simulink model "EPT"  (R2019b)
settings: Solver=FixedStepDiscrete  StartTime=0.0  StopTime=5  FixedStep=0.005  RelTol=1e-3  EnableMultiTasking=on
PreLoadFcn:
  | try, model_open; catch, disp('Error occurred while executing model pre-load callback: model_open.m'); disp('Please assure that the MATLAB working directory is set to the model directory before opening.'); end
InitFcn:
  | try, model_open; catch, end
undefined symbols (not defined in the file or in its folder): Bridge, GCM, H, ln, raptor_get_param_eval, raptor_get_safe_string, raptor_xcp_function
libraries: Raptor_lib x2810, simulink x374, hdlsllib x19
(part 3 of 45)

== system EPT/Foreground_TimeBase_5ms/CHG//DCHG_PW_Control/Batt_Temperature Coefficient ==
  Compare To Constant : simulink/Logic and Bit Operations/Compare To Constant  relop=<  const=20  OutDataTypeStr=boolean
  Compare To Constant1 : simulink/Logic and Bit Operations/Compare To Constant  relop=<  const=35  OutDataTypeStr=boolean
  Constant4 : Constant
  Constant5 : Constant
  Demux1 : Demux  Outputs=2
  Max : MinMax  Function=max  Inputs=2
  MinMax : MinMax  Inputs=2
  Mux1 : Mux  Inputs=2
  Product1 : Product
  Saturation : Saturate  UpperLimit=60  LowerLimit=-10
  Saturation1 : Saturate  UpperLimit=60  LowerLimit=-10
  Switch : Switch  Criteria=u2 > Threshold
  Switch1 : Switch  Criteria=u2 > Threshold
  raptor_data_def1 : Raptor_lib/Data Storage/raptor_data_def  dataName='Max_CellT'  initValue=0  dataType=double  storage=Volatile (RAM)  calVisible=on  calType=Measurement  calDispType=Number  calEnum={'False', 'True'}  calGain=1.0  calOffset=0  calMin=-inf  calMax=inf  calFormat='-1'  calUnit=''  calHelp=''  calAccess=1  calFunction=raptor_xcp_function(gcb)  calDispHeaders=off  calColHeaders={'Col1' 'Col2' 'Col3'}  calRowHeaders={'Row1' 'Row2' 'Row3'}
      settings: SourceProductName=Raptor
  raptor_data_def2 : Raptor_lib/Data Storage/raptor_data_def  dataName='Min_CellT'  initValue=0  dataType=double  storage=Volatile (RAM)  calVisible=on  calType=Measurement  calDispType=Number  calEnum={'False', 'True'}  calGain=1.0  calOffset=0  calMin=-inf  calMax=inf  calFormat='-1'  calUnit=''  calHelp=''  calAccess=1  calFunction=raptor_xcp_function(gcb)  calDispHeaders=off  calColHeaders={'Col1' 'Col2' 'Col3'}  calRowHeaders={'Row1' 'Row2' 'Row3'}
      settings: SourceProductName=Raptor
  raptor_data_read1 : Raptor_lib/Data Storage/raptor_data_read  dataName='CMU1_CELL_TEMP_MIN'  dataShape=Scalar  idxSource=Input  idxRow=1  idxCol=1
      settings: SourceProductName=Raptor
  raptor_data_read2 : Raptor_lib/Data Storage/raptor_data_read  dataName='CMU2_CELL_TEMP_MIN'  dataShape=Scalar  idxSource=Input  idxRow=1  idxCol=1
      settings: SourceProductName=Raptor
  raptor_data_read3 : Raptor_lib/Data Storage/raptor_data_read  dataName='CMU2_CELL_TEMP_MAX'  dataShape=Scalar  idxSource=Input  idxRow=1  idxCol=1
      settings: SourceProductName=Raptor
  raptor_data_read7 : Raptor_lib/Data Storage/raptor_data_read  dataName='CMU1_CELL_TEMP_MAX'  dataShape=Scalar  idxSource=Input  idxRow=1  idxCol=1
      settings: SourceProductName=Raptor
  raptor_data_write : Raptor_lib/Data Storage/raptor_data_write  dataName='Min_CellT'  dataShape=Scalar  idxSource=Input Port  idxRow=1  idxCol=1
      settings: SourceProductName=Raptor
  raptor_data_write1 : Raptor_lib/Data Storage/raptor_data_write  dataName='Max_CellT'  dataShape=Scalar  idxSource=Input Port  idxRow=1  idxCol=1
      settings: SourceProductName=Raptor
  raptor_measurement4 : Raptor_lib/Data Storage/raptor_measurement  paramName='Ft'  nameSource=Parameter  calDispType=Number  calEnum={'False', 'True'}  calGain=1.0  calOffset=0.0  calMax=inf  calMin=-inf  calFormat='-1'  calUnit=''  calHelp=''  calAccess=1  calFunction=raptor_xcp_function(gcb)  calVisible=on
      settings: SourceProductName=Raptor
  raptor_override1 : Raptor_lib/Data Storage/raptor_override  paramName='Cal_Min_CellT'  nameSource=Parameter  measurement=None  calDispType=Number  calEnum={'False', 'True'}  calGain=1.0  calOffset=0.0  calMax=inf  calMin=-inf  calFormat='-1'  calUnit=''  calHelp=''  calAccess=1  calFunction=[raptor_xcp_function(gcb) '|' raptor_get_param_eval(gcb, 'paramName') '_Override']
      settings: SourceProductName=Raptor
  raptor_override5 : Raptor_lib/Data Storage/raptor_override  paramName='Cal_Max_CellT'  nameSource=Parameter  measurement=None  calDispType=Number  calEnum={'False', 'True'}  calGain=1.0  calOffset=0.0  calMax=inf  calMin=-inf  calFormat='-1'  calUnit=''  calHelp=''  calAccess=1  calFunction=[raptor_xcp_function(gcb) '|' raptor_get_param_eval(gcb, 'paramName') '_Override']
      settings: SourceProductName=Raptor
  raptor_table_1d3 : Raptor_lib/Table Lookup/raptor_table_1d  dataName='Temp2Ft'  initValue="[0.1\t0.2\t0.5\t0.8\t0.9\t1\t1\t1\t0.8\t0.6\t0.4\t0.2\t0.1]"  dataType=double  storage=Calibration  initValueX="[60\t55\t50\t45\t40\t35\t25\t20\t10\t5\t0\t-5\t-10]"  dataTypeXY=double  storageXY=Calibration  calVisible=on  showTable=on  calGain=1.0  calOffset=0.0  calMax=Inf  calMin=-Inf  calFormat='-1'  calUnit=''  calHelp=''  showBreakpoint=on  dataNameX=[]  calGainX=1.0  calOffsetX=0.0  calMaxX=Inf  calMinX=-Inf  calFormatX='-1'  calUnitX=''  calHelpX=''  calAccess=1  calFunction=raptor_xcp_function(gcb)  measureEnable=off  mName=[raptor_get_param_eval(gcb,'dataName'), '_Output']
      settings: SourceProductName=Raptor
  Ft : Outport  VectorParamsAs1DForOutWhenUnconnected=off
  wires:
  Compare To Constant1/1 -> Switch/2
  Switch/1 -> Product1/1
  Demux1/2 -> Switch1/1
  Constant4/1 -> Switch/1
  Product1/1 -> Ft/1, raptor_measurement4/1
  Max/1 -> raptor_override5/1
  Compare To Constant/1 -> Switch1/2
  Demux1/1 -> Switch/3
  Mux1/1 -> raptor_table_1d3/1
  raptor_data_read7/1 -> Max/1
  raptor_data_read1/1 -> MinMax/1
  raptor_table_1d3/1 -> Demux1/1
  Switch1/1 -> Product1/2
  Constant5/1 -> Switch1/3
  Saturation/1 -> Compare To Constant1/1, Mux1/1
  Saturation1/1 -> Mux1/2, Compare To Constant/1
  raptor_data_read3/1 -> Max/2
  raptor_data_read2/1 -> MinMax/2
  MinMax/1 -> raptor_override1/1
  raptor_override5/1 -> raptor_data_write1/1, Saturation/1
  raptor_override1/1 -> raptor_data_write/1, Saturation1/1

== system EPT/Foreground_TimeBase_5ms/CHG//DCHG_PW_Control/CHG//DCHG_Current_Control ==
  Ft : Inport
  Constant : Constant
  Idchg_con Soft Recovery : Subsystem
  "Idchg_con Soft Recovery " : Subsystem  Commented=on
  Max2 : MinMax  Function=max  Inputs=2
  Min1 : MinMax  Inputs=2
  Min2 : MinMax  Inputs=2
  Product : Product  Inputs=3
  Product{2..5} (4 alike) : Product
  Saturation Dynamic1 : simulink/Discontinuities/Saturation Dynamic  OutMin=[]  OutMax=[]  OutDataTypeStr=Inherit: Same as second input  OutDataType=fixdt(1, 16)  OutScaling=2^-10  DoSatur=off
  Soft Recovery : Subsystem
  Switch{,1..4} (5 alike) : Switch  Criteria=u2 > Threshold
  raptor_adjustment1 : Raptor_lib/Data Storage/raptor_adjustment  paramName='Cal_CHG_Max_Current'  nameSource=Parameter  initValue=30  dataType=double  storage=Calibration  calDispType=Number  calEnum={'False', 'True'}  calGain=1.0  calOffset=0.0  calMax=inf  calMin=-inf  calFormat='-1'  calUnit=''  calHelp=''  calAccess=1  calFunction=raptor_xcp_function(gcb)  calDispHeaders=off  calColHeaders={'Col1' 'Col2' 'Col3'}  calRowHeaders={'Row1' 'Row2' 'Row3'}
      settings: SourceProductName=Raptor
  raptor_adjustment2 : Raptor_lib/Data Storage/raptor_adjustment  paramName='Cal_Vcell_Decline_Ft'  nameSource=Parameter  initValue=1  dataType=double  storage=Calibration  calDispType=Number  calEnum={'False', 'True'}  calGain=1.0  calOffset=0.0  calMax=inf  calMin=-inf  calFormat='-1'  calUnit=''  calHelp=''  calAccess=1  calFunction=raptor_xcp_function(gcb)  calDispHeaders=off  calColHeaders={'Col1' 'Col2' 'Col3'}  calRowHeaders={'Row1' 'Row2' 'Row3'}
      settings: SourceProductName=Raptor
  raptor_adjustment3 : Raptor_lib/Data Storage/raptor_adjustment  paramName='Cal_Ichg_cc_Exp_Max'  nameSource=Parameter  initValue=100  dataType=double  storage=Calibration  calDispType=Number  calEnum={'False', 'True'}  calGain=1.0  calOffset=0.0  calMax=inf  calMin=-inf  calFormat='-1'  calUnit=''  calHelp=''  calAccess=1  calFunction=raptor_xcp_function(gcb)  calDispHeaders=off  calColHeaders={'Col1' 'Col2' 'Col3'}  calRowHeaders={'Row1' 'Row2' 'Row3'}
      settings: SourceProductName=Raptor
  raptor_adjustment4 : Raptor_lib/Data Storage/raptor_adjustment  paramName='Cal_Ichg_cc_Exp_Min'  nameSource=Parameter  initValue=15  dataType=double  storage=Calibration  calDispType=Number  calEnum={'False', 'True'}  calGain=1.0  calOffset=0.0  calMax=inf  calMin=-inf  calFormat='-1'  calUnit=''  calHelp=''  calAccess=1  calFunction=raptor_xcp_function(gcb)  calDispHeaders=off  calColHeaders={'Col1' 'Col2' 'Col3'}  calRowHeaders={'Row1' 'Row2' 'Row3'}
      settings: SourceProductName=Raptor
  raptor_adjustment5 : Raptor_lib/Data Storage/raptor_adjustment  paramName='Cal_Idchg_con_Source'  nameSource=Parameter  initValue=0  dataType=boolean  storage=Calibration  calDispType=Number  calEnum={'False', 'True'}  calGain=1.0  calOffset=0.0  calMax=inf  calMin=-inf  calFormat='-1'  calUnit=''  calHelp=''  calAccess=1  calFunction=raptor_xcp_function(gcb)  calDispHeaders=off  calColHeaders={'Col1' 'Col2' 'Col3'}  calRowHeaders={'Row1' 'Row2' 'Row3'}
      settings: SourceProductName=Raptor
  raptor_adjustment6 : Raptor_lib/Data Storage/raptor_adjustment  paramName='Cal_Idchg_exp_Source'  nameSource=Parameter  initValue=0  dataType=boolean  storage=Calibration  calDispType=Number  calEnum={'False', 'True'}  calGain=1.0  calOffset=0.0  calMax=inf  calMin=-inf  calFormat='-1'  calUnit=''  calHelp=''  calAccess=1  calFunction=raptor_xcp_function(gcb)  calDispHeaders=off  calColHeaders={'Col1' 'Col2' 'Col3'}  calRowHeaders={'Row1' 'Row2' 'Row3'}
      settings: SourceProductName=Raptor
  raptor_data_def : Raptor_lib/Data Storage/raptor_data_def  dataName='Ichg_cc_exp'  initValue=0  dataType=double  storage=Volatile (RAM)  calVisible=on  calType=Measurement  calDispType=Number  calEnum={'False', 'True'}  calGain=1.0  calOffset=0  calMin=-inf  calMax=inf  calFormat='-1'  calUnit=''  calHelp=''  calAccess=1  calFunction=raptor_xcp_function(gcb)  calDispHeaders=off  calColHeaders={'Col1' 'Col2' 'Col3'}  calRowHeaders={'Row1' 'Row2' 'Row3'}
      settings: SourceProductName=Raptor
  raptor_data_def1 : Raptor_lib/Data Storage/raptor_data_def  dataName='Idchg_con_exp'  initValue=0  dataType=double  storage=Volatile (RAM)  calVisible=on  calType=Measurement  calDispType=Number  calEnum={'False', 'True'}  calGain=1.0  calOffset=0  calMin=-inf  calMax=inf  calFormat='-1'  calUnit=''  calHelp=''  calAccess=1  calFunction=raptor_xcp_function(gcb)  calDispHeaders=off  calColHeaders={'Col1' 'Col2' 'Col3'}  calRowHeaders={'Row1' 'Row2' 'Row3'}
      settings: SourceProductName=Raptor
  raptor_data_def2 : Raptor_lib/Data Storage/raptor_data_def  dataName='Max_CellV'  initValue=0  dataType=double  storage=Volatile (RAM)  calVisible=on  calType=Adjustment  calDispType=Number  calEnum={'False', 'True'}  calGain=1.0  calOffset=0  calMin=-inf  calMax=inf  calFormat='2.3'  calUnit=''  calHelp=''  calAccess=1  calFunction=raptor_xcp_function(gcb)  calDispHeaders=off  calColHeaders={'Col1' 'Col2' 'Col3'}  calRowHeaders={'Row1' 'Row2' 'Row3'}
      settings: SourceProductName=Raptor
  raptor_data_def3 : Raptor_lib/Data Storage/raptor_data_def  dataName='Min_CellV'  initValue=0  dataType=double  storage=Volatile (RAM)  calVisible=on  calType=Adjustment  calDispType=Number  calEnum={'False', 'True'}  calGain=1.0  calOffset=0  calMin=-inf  calMax=inf  calFormat='2.3'  calUnit=''  calHelp=''  calAccess=1  calFunction=raptor_xcp_function(gcb)  calDispHeaders=off  calColHeaders={'Col1' 'Col2' 'Col3'}  calRowHeaders={'Row1' 'Row2' 'Row3'}
      settings: SourceProductName=Raptor
  raptor_data_def4 : Raptor_lib/Data Storage/raptor_data_def  dataName='Iregen_con_exp'  initValue=0  dataType=double  storage=Volatile (RAM)  calVisible=on  calType=Measurement  calDispType=Number  calEnum={'False', 'True'}  calGain=1.0  calOffset=0  calMin=-inf  calMax=inf  calFormat='-1'  calUnit=''  calHelp=''  calAccess=1  calFunction=raptor_xcp_function(gcb)  calDispHeaders=off  calColHeaders={'Col1' 'Col2' 'Col3'}  calRowHeaders={'Row1' 'Row2' 'Row3'}
      settings: SourceProductName=Raptor
  raptor_data_def5 : Raptor_lib/Data Storage/raptor_data_def  dataName='Idchg_con'  initValue=0  dataType=double  storage=Volatile (RAM)  calVisible=on  calType=Measurement  calDispType=Number  calEnum={'False', 'True'}  calGain=1.0  calOffset=0  calMin=-inf  calMax=inf  calFormat='-1'  calUnit=''  calHelp=''  calAccess=1  calFunction=raptor_xcp_function(gcb)  calDispHeaders=off  calColHeaders={'Col1' 'Col2' 'Col3'}  calRowHeaders={'Row1' 'Row2' 'Row3'}
      settings: SourceProductName=Raptor
  raptor_data_def6 : Raptor_lib/Data Storage/raptor_data_def  dataName='Ft_CHG_Vcell'  initValue=0  dataType=double  storage=Volatile (RAM)  calVisible=on  calType=Adjustment  calDispType=Number  calEnum={'False', 'True'}  calGain=1.0  calOffset=0  calMin=-inf  calMax=inf  calFormat='2.3'  calUnit=''  calHelp=''  calAccess=1  calFunction=raptor_xcp_function(gcb)  calDispHeaders=off  calColHeaders={'Col1' 'Col2' 'Col3'}  calRowHeaders={'Row1' 'Row2' 'Row3'}
      settings: SourceProductName=Raptor
  raptor_data_read1 : Raptor_lib/Data Storage/raptor_data_read  dataName='EPT_BPOBU_SOC'  dataShape=Scalar  idxSource=Input  idxRow=1  idxCol=1
      settings: SourceProductName=Raptor
  raptor_data_read2 : Raptor_lib/Data Storage/raptor_data_read  dataName='Read_OBC_Temp'  dataShape=Scalar  idxSource=Input  idxRow=1  idxCol=1
      settings: SourceProductName=Raptor
  raptor_data_read3 : Raptor_lib/Data Storage/raptor_data_read  dataName='CMU2_CELL_VOLT_MAX'  dataShape=Scalar  idxSource=Input  idxRow=1  idxCol=1
      settings: SourceProductName=Raptor
  raptor_data_read4 : Raptor_lib/Data Storage/raptor_data_read  dataName='CMU1_CELL_VOLT_MAX'  dataShape=Scalar  idxSource=Input  idxRow=1  idxCol=1
      settings: SourceProductName=Raptor
  raptor_data_read5 : Raptor_lib/Data Storage/raptor_data_read  dataName='CMU2_CELL_VOLT_MIN'  dataShape=Scalar  idxSource=Input  idxRow=1  idxCol=1
      settings: SourceProductName=Raptor
  raptor_data_read6 : Raptor_lib/Data Storage/raptor_data_read  dataName='CMU1_CELL_VOLT_MIN'  dataShape=Scalar  idxSource=Input  idxRow=1  idxCol=1
      settings: SourceProductName=Raptor
  raptor_data_read7 : Raptor_lib/Data Storage/raptor_data_read  dataName='Flag_CHG_Mode'  dataShape=Scalar  idxSource=Input  idxRow=1  idxCol=1
      settings: SourceProductName=Raptor
  raptor_data_read8 : Raptor_lib/Data Storage/raptor_data_read  dataName='Flag_Drive_Mode'  dataShape=Scalar  idxSource=Input  idxRow=1  idxCol=1
      settings: SourceProductName=Raptor
  raptor_data_read9 : Raptor_lib/Data Storage/raptor_data_read  dataName='EPT_BPOBU_CURR'  dataShape=Scalar  idxSource=Input  idxRow=1  idxCol=1
      settings: SourceProductName=Raptor
  raptor_data_write : Raptor_lib/Data Storage/raptor_data_write  dataName='Ichg_cc_exp'  dataShape=Scalar  idxSource=Input Port  idxRow=1  idxCol=1
      settings: SourceProductName=Raptor
  raptor_data_write1 : Raptor_lib/Data Storage/raptor_data_write  dataName='Idchg_con_exp'  dataShape=Scalar  idxSource=Input Port  idxRow=1  idxCol=1
      settings: SourceProductName=Raptor
  raptor_data_write2 : Raptor_lib/Data Storage/raptor_data_write  dataName='Min_CellV'  dataShape=Scalar  idxSource=Input Port  idxRow=1  idxCol=1
      settings: SourceProductName=Raptor
  raptor_data_write3 : Raptor_lib/Data Storage/raptor_data_write  dataName='Max_CellV'  dataShape=Scalar  idxSource=Input Port  idxRow=1  idxCol=1
      settings: SourceProductName=Raptor
  raptor_data_write4 : Raptor_lib/Data Storage/raptor_data_write  dataName='Iregen_con_exp'  dataShape=Scalar  idxSource=Input Port  idxRow=1  idxCol=1
      settings: SourceProductName=Raptor
  raptor_data_write5 : Raptor_lib/Data Storage/raptor_data_write  dataName='Idchg_con'  dataShape=Scalar  idxSource=Input Port  idxRow=1  idxCol=1
      settings: SourceProductName=Raptor
  raptor_data_write6 : Raptor_lib/Data Storage/raptor_data_write  dataName='Ft_CHG_Vcell'  dataShape=Scalar  idxSource=Input Port  idxRow=1  idxCol=1
      settings: SourceProductName=Raptor
  raptor_override : Raptor_lib/Data Storage/raptor_override  paramName='Cal_Idchg_con_exp'  nameSource=Parameter  measurement=None  calDispType=Number  calEnum={'False', 'True'}  calGain=1.0  calOffset=0.0  calMax=inf  calMin=-inf  calFormat='-1'  calUnit=''  calHelp=''  calAccess=1  calFunction=[raptor_xcp_function(gcb) '|' raptor_get_param_eval(gcb, 'paramName') '_Override']
      settings: SourceProductName=Raptor
  raptor_override1 : Raptor_lib/Data Storage/raptor_override  paramName='Cal_Ichg_cc_exp'  nameSource=Parameter  measurement=None  calDispType=Number  calEnum={'False', 'True'}  calGain=1.0  calOffset=0.0  calMax=inf  calMin=-inf  calFormat='-1'  calUnit=''  calHelp=''  calAccess=1  calFunction=[raptor_xcp_function(gcb) '|' raptor_get_param_eval(gcb, 'paramName') '_Override']
      settings: SourceProductName=Raptor
  raptor_override2 : Raptor_lib/Data Storage/raptor_override  paramName='Cal_CHGERTemp2Ft'  nameSource=Parameter  measurement=None  calDispType=Number  calEnum={'False', 'True'}  calGain=1.0  calOffset=0.0  calMax=inf  calMin=-inf  calFormat='-1'  calUnit=''  calHelp=''  calAccess=1  calFunction=[raptor_xcp_function(gcb) '|' raptor_get_param_eval(gcb, 'paramName') '_Override']
      settings: SourceProductName=Raptor
  raptor_override3 : Raptor_lib/Data Storage/raptor_override  paramName='Cal_Idchg_con'  nameSource=Parameter  measurement=None  calDispType=Number  calEnum={'False', 'True'}  calGain=1.0  calOffset=0.0  calMax=inf  calMin=-inf  calFormat='-1'  calUnit=''  calHelp=''  calAccess=1  calFunction=[raptor_xcp_function(gcb) '|' raptor_get_param_eval(gcb, 'paramName') '_Override']
      settings: SourceProductName=Raptor
  raptor_override4 : Raptor_lib/Data Storage/raptor_override  paramName='Cal_Min_CellV'  nameSource=Parameter  measurement=None  calDispType=Number  calEnum={'False', 'True'}  calGain=1.0  calOffset=0.0  calMax=inf  calMin=-inf  calFormat='-1'  calUnit=''  calHelp=''  calAccess=1  calFunction=[raptor_xcp_function(gcb) '|' raptor_get_param_eval(gcb, 'paramName') '_Override']
      settings: SourceProductName=Raptor
  raptor_override5 : Raptor_lib/Data Storage/raptor_override  paramName='Cal_Max_CellV'  nameSource=Parameter  measurement=None  calDispType=Number  calEnum={'False', 'True'}  calGain=1.0  calOffset=0.0  calMax=inf  calMin=-inf  calFormat='-1'  calUnit=''  calHelp=''  calAccess=1  calFunction=[raptor_xcp_function(gcb) '|' raptor_get_param_eval(gcb, 'paramName') '_Override']
      settings: SourceProductName=Raptor
  raptor_table_1d1 : Raptor_lib/Table Lookup/raptor_table_1d  dataName='Remaining_Capability2Idchg_con'  initValue="[-50\t-100\t-150\t-250\t-300\t-300\t-300\t-300\t-300\t-300\t-300\t-300\t-300]"  dataType=double  storage=Calibration  initValueX="[0\t10\t18\t26\t34\t42\t50\t58\t66\t74\t82\t90\t100]"  dataTypeXY=double  storageXY=Calibration  calVisible=on  showTable=on  calGain=1.0  calOffset=0.0  calMax=Inf  calMin=-Inf  calFormat='-1'  calUnit=''  calHelp=''  showBreakpoint=on  dataNameX=[]  calGainX=1.0  calOffsetX=0.0  calMaxX=Inf  calMinX=-Inf  calFormatX='-1'  calUnitX=''  calHelpX=''  calAccess=1  calFunction=raptor_xcp_function(gcb)  measureEnable=off  mName=[raptor_get_param_eval(gcb,'dataName'), '_Output']
      settings: SourceProductName=Raptor
  raptor_table_1d2 : Raptor_lib/Table Lookup/raptor_table_1d  dataName='Remaining_Capability2Ichg_cc'  initValue="[50\t50\t75\t75\t75\t75\t75\t75\t75\t75\t50\t30\t15]"  dataType=double  storage=Calibration  initValueX="[0\t10\t18\t26\t34\t42\t50\t58\t66\t74\t82\t90\t100]"  dataTypeXY=double  storageXY=Calibration  calVisible=on  showTable=on  calGain=1.0  calOffset=0.0  calMax=Inf  calMin=-Inf  calFormat='-1'  calUnit=''  calHelp=''  showBreakpoint=on  dataNameX=[]  calGainX=1.0  calOffsetX=0.0  calMaxX=Inf  calMinX=-Inf  calFormatX='-1'  calUnitX=''  calHelpX=''  calAccess=1  calFunction=raptor_xcp_function(gcb)  measureEnable=off  mName=[raptor_get_param_eval(gcb,'dataName'), '_Output']
      settings: SourceProductName=Raptor
  raptor_table_1d3 : Raptor_lib/Table Lookup/raptor_table_1d  dataName='CHGTemp2Ft'  initValue=[0.5,0.75,1,1,1,1,1,1,0.8,0.3,0.10,0,0.0,0]  dataType=double  storage=Calibration  initValueX=[-40,-20,-10,0,10,20,30,50,56,58,60,65,70,80]  dataTypeXY=double  storageXY=Calibration  calVisible=on  showTable=on  calGain=1.0  calOffset=0.0  calMax=Inf  calMin=-Inf  calFormat='-1'  calUnit=''  calHelp=''  showBreakpoint=on  dataNameX=[]  calGainX=1.0  calOffsetX=0.0  calMaxX=Inf  calMinX=-Inf  calFormatX='-1'  calUnitX=''  calHelpX=''  calAccess=1  calFunction=raptor_xcp_function(gcb)  measureEnable=off  mName=[raptor_get_param_eval(gcb,'dataName'), '_Output']
      settings: SourceProductName=Raptor
  raptor_table_1d4 : Raptor_lib/Table Lookup/raptor_table_1d  dataName='Vcell2CHG_Ft'  initValue=[1,1,0.2,0.2,0.1]  dataType=double  storage=Calibration  initValueX=[3.4,3.45,3.5,3.55,3.6]  dataTypeXY=double  storageXY=Calibration  calVisible=on  showTable=on  calGain=1.0  calOffset=0.0  calMax=Inf  calMin=-Inf  calFormat='-1'  calUnit=''  calHelp=''  showBreakpoint=on  dataNameX=[]  calGainX=1.0  calOffsetX=0.0  calMaxX=Inf  calMinX=-Inf  calFormatX='-1'  calUnitX=''  calHelpX=''  calAccess=1  calFunction=raptor_xcp_function(gcb)  measureEnable=off  mName=[raptor_get_param_eval(gcb,'dataName'), '_Output']
      settings: SourceProductName=Raptor
  raptor_table_1d6 : Raptor_lib/Table Lookup/raptor_table_1d  dataName='Remaining_Capability2Iregen_con'  initValue=|  dataType=double  storage=Calibration  initValueX="[0\t10\t18\t26\t34\t42\t50\t58\t66\t74\t82\t90\t100]"  dataTypeXY=double  storageXY=Calibration  calVisible=on  showTable=on  calGain=1.0  calOffset=0.0  calMax=Inf  calMin=-Inf  calFormat='-1'  calUnit=''  calHelp=''  showBreakpoint=on  dataNameX=[]  calGainX=1.0  calOffsetX=0.0  calMaxX=Inf  calMinX=-Inf  calFormatX='-1'  calUnitX=''  calHelpX=''  calAccess=1  calFunction=raptor_xcp_function(gcb)  measureEnable=off  mName=[raptor_get_param_eval(gcb,'dataName'), '_Output']
      | [50
      | 100
      | 150
      | 150
      | 150
      | 150
      | 150
      | 150
      | 150
      | 100
      | 50
      | 30
      | 15
      | ]
      settings: SourceProductName=Raptor
  raptor_table_1d8 : Raptor_lib/Table Lookup/raptor_table_1d  dataName='Vcell2DisCHG_Ft'  initValue=[1,1,1,0.1]  dataType=double  storage=Calibration  initValueX=[3.6,3.1,2.8,2.5]  dataTypeXY=double  storageXY=Calibration  calVisible=on  showTable=on  calGain=1.0  calOffset=0.0  calMax=Inf  calMin=-Inf  calFormat='-1'  calUnit=''  calHelp=''  showBreakpoint=on  dataNameX=[]  calGainX=1.0  calOffsetX=0.0  calMaxX=Inf  calMinX=-Inf  calFormatX='-1'  calUnitX=''  calHelpX=''  calAccess=1  calFunction=raptor_xcp_function(gcb)  measureEnable=off  mName=[raptor_get_param_eval(gcb,'dataName'), '_Output']
      settings: SourceProductName=Raptor
  Idchg_exp : Outport  VectorParamsAs1DForOutWhenUnconnected=off
  Iregen_con : Outport  Port=2  VectorParamsAs1DForOutWhenUnconnected=off
  wires:
  raptor_table_1d1/1 -> Product/2
  raptor_data_read1/1 -> raptor_table_1d6/1, raptor_table_1d1/1, raptor_table_1d2/1
  raptor_table_1d2/1 -> Product2/2
  raptor_data_read2/1 -> raptor_table_1d3/1
  Product2/1 -> Product3/1
  raptor_data_read4/1 -> Max2/1
  raptor_data_read3/1 -> Max2/2
  Max2/1 -> raptor_override5/1
  raptor_data_read6/1 -> Min1/1
  raptor_data_read5/1 -> Min1/2
  Min1/1 -> raptor_override4/1
  Switch/1 -> raptor_data_write6/1, Product3/2
  raptor_table_1d4/1 -> Switch/1
  Constant/1 -> Switch/3
  raptor_adjustment2/1 -> Switch/2
  raptor_adjustment1/1 -> Product4/1
  raptor_table_1d3/1 -> raptor_override2/1
  raptor_adjustment3/1 -> Saturation Dynamic1/1, Switch2/1
  Product4/1 -> Min2/2
  Product3/1 -> Min2/1
  Product5/1 -> raptor_data_write4/1, Iregen_con/1
  Ft/1 -> Product5/1, Product2/1, Product/3
  raptor_table_1d6/1 -> Product5/2
  raptor_table_1d8/1 -> Product/1
  Switch4/1 -> Idchg_exp/1, raptor_data_write1/1
  raptor_override1/1 -> raptor_data_write/1
  raptor_override2/1 -> Product4/2
  Product/1 -> Idchg_con Soft Recovery/1(Idchg_con_input), Switch3/1
  raptor_data_read9/1 -> Soft Recovery/1(HV_Current)
  Soft Recovery/1(Idchg_exp) -> raptor_override/1
  Min2/1 -> Switch1/3, Saturation Dynamic1/2
  raptor_adjustment4/1 -> Saturation Dynamic1/3
  raptor_override3/1 -> Switch4/3, raptor_data_write5/1, Soft Recovery/2(Idchg_con)
  Saturation Dynamic1/1 -> Switch1/1
  Switch2/1 -> raptor_override1/1
  raptor_data_read7/1 -> Switch1/2
  raptor_data_read8/1 -> Switch2/2
  Switch1/1 -> Switch2/3
  raptor_override4/1 -> raptor_table_1d8/1, raptor_data_write2/1
  raptor_override5/1 -> raptor_data_write3/1, raptor_table_1d4/1
  Idchg_con Soft Recovery/1(Idchg_con_output) -> Switch3/3
  Switch3/1 -> raptor_override3/1
  raptor_adjustment5/1 -> Switch3/2
  raptor_override/1 -> Switch4/1
  raptor_adjustment6/1 -> Switch4/2

== system EPT/Foreground_TimeBase_5ms/CHG//DCHG_PW_Control/Coulomb Counting Algorithm ==
  note: Notes:
      | CMU	:0
      | EPT   	:1
  Abs : Abs
  Add3 : Sum
  Compare To Constant1 : simulink/Logic and Bit Operations/Compare To Constant  relop=>  const=500  OutDataTypeStr=boolean
  Compare To Zero : simulink/Logic and Bit Operations/Compare To Zero  relop=<=  OutDataTypeStr=boolean
  Constant1 : Constant  Value=400
  Coulomb Counting Algorithm : Subsystem
  Delay : Subsystem
  Divide : Product  Inputs=*/
  Divide1 : Product  Inputs=*/
  Gain1 : Gain  Gain=100
  Gain3 : Gain  Gain=100
  Gain4 : Gain  Gain=0.5
  Latch : Subsystem
  Logical Operator1 : Logic  Inputs=3  AllPortsSameDT=off  OutDataTypeStr=boolean
  NOT : Logic  Operator=NOT  IconShape=distinctive  AllPortsSameDT=off  OutDataTypeStr=boolean
  NOT1 : Logic  Operator=NOT  IconShape=distinctive  AllPortsSameDT=off  OutDataTypeStr=boolean
  NOT2 : Logic  Operator=NOT  IconShape=distinctive  AllPortsSameDT=off  OutDataTypeStr=boolean
  Switch1 : Switch  Criteria=u2 > Threshold
  Switch4 : Switch  Criteria=u2 > Threshold
  "WH " : Subsystem
  raptor_adjustment1 : Raptor_lib/Data Storage/raptor_adjustment  paramName='Cal_BP_OBU_AH_Def'  nameSource=Parameter  initValue=135  dataType=uint8  storage=Calibration  calDispType=Number  calEnum={'False', 'True'}  calGain=1.0  calOffset=0.0  calMax=inf  calMin=-inf  calFormat='-1'  calUnit=''  calHelp=''  calAccess=1  calFunction=raptor_xcp_function(gcb)  calDispHeaders=off  calColHeaders={'Col1' 'Col2' 'Col3'}  calRowHeaders={'Row1' 'Row2' 'Row3'}
      settings: SourceProductName=Raptor
  raptor_adjustment2 : Raptor_lib/Data Storage/raptor_adjustment  paramName='Cal_RSOC_Resource'  nameSource=Parameter  initValue=1  dataType=boolean  storage=Calibration  calDispType=Number  calEnum={'False', 'True'}  calGain=1.0  calOffset=0.0  calMax=inf  calMin=-inf  calFormat='-1'  calUnit=''  calHelp=''  calAccess=1  calFunction=raptor_xcp_function(gcb)  calDispHeaders=off  calColHeaders={'Col1' 'Col2' 'Col3'}  calRowHeaders={'Row1' 'Row2' 'Row3'}
      settings: SourceProductName=Raptor
  raptor_data_read14 : Raptor_lib/Data Storage/raptor_data_read  dataName='EPT_BPOBU_FCCAP'  dataShape=Scalar  idxSource=Input  idxRow=1  idxCol=1
      settings: SourceProductName=Raptor
  raptor_data_read15 : Raptor_lib/Data Storage/raptor_data_read  dataName='CAN_Fault_CMU1'  dataShape=Scalar  idxSource=Input  idxRow=1  idxCol=1
      settings: SourceProductName=Raptor
  raptor_data_read16 : Raptor_lib/Data Storage/raptor_data_read  dataName='EPT_BPOBU_CURR'  dataShape=Scalar  idxSource=Input  idxRow=1  idxCol=1
      settings: SourceProductName=Raptor
  raptor_data_read17 : Raptor_lib/Data Storage/raptor_data_read  dataName='EPT_BPOBU_RCAP'  dataShape=Scalar  idxSource=Input  idxRow=1  idxCol=1
      settings: SourceProductName=Raptor
  raptor_data_read18 : Raptor_lib/Data Storage/raptor_data_read  dataName='CMU2_REMAIN_CAPACITY'  dataShape=Scalar  idxSource=Input  idxRow=1  idxCol=1
      settings: SourceProductName=Raptor
  raptor_data_read19 : Raptor_lib/Data Storage/raptor_data_read  dataName='CMU1_REMAIN_CAPACITY'  dataShape=Scalar  idxSource=Input  idxRow=1  idxCol=1
      settings: SourceProductName=Raptor
  raptor_data_read20 : Raptor_lib/Data Storage/raptor_data_read  dataName='EPT_BPOBU_VOLT'  dataShape=Scalar  idxSource=Input  idxRow=1  idxCol=1
      settings: SourceProductName=Raptor
  raptor_data_read21 : Raptor_lib/Data Storage/raptor_data_read  dataName='EPT_CONSUMED_WH'  dataShape=Scalar  idxSource=Input  idxRow=1  idxCol=1
      settings: SourceProductName=Raptor
  raptor_data_read22 : Raptor_lib/Data Storage/raptor_data_read  dataName='CAN_Fault_CMU2'  dataShape=Scalar  idxSource=Input  idxRow=1  idxCol=1
      settings: SourceProductName=Raptor
  raptor_data_read3 : Raptor_lib/Data Storage/raptor_data_read  dataName='EPT_BPOBU_FCCAP'  dataShape=Scalar  idxSource=Input  idxRow=1  idxCol=1
      settings: SourceProductName=Raptor
  raptor_data_write : Raptor_lib/Data Storage/raptor_data_write  dataName='EPT_BPOBU_AH_DEF'  dataShape=Scalar  idxSource=Input Port  idxRow=1  idxCol=1
      settings: SourceProductName=Raptor
  raptor_data_write6 : Raptor_lib/Data Storage/raptor_data_write  dataName='EPT_BPOBU_SOC'  dataShape=Scalar  idxSource=Input Port  idxRow=1  idxCol=1
      settings: SourceProductName=Raptor
  raptor_data_write7 : Raptor_lib/Data Storage/raptor_data_write  dataName='EPT_BPOBU_SOA'  dataShape=Scalar  idxSource=Input Port  idxRow=1  idxCol=1
      settings: SourceProductName=Raptor
  raptor_data_write8 : Raptor_lib/Data Storage/raptor_data_write  dataName='EPT_CONSUMED_WH'  dataShape=Scalar  idxSource=Input Port  idxRow=1  idxCol=1
      settings: SourceProductName=Raptor
  raptor_override2 : Raptor_lib/Data Storage/raptor_override  paramName='Cal_EPT_CONSUMED_WH'  nameSource=Parameter  measurement=None  calDispType=Number  calEnum={'False', 'True'}  calGain=1.0  calOffset=0.0  calMax=inf  calMin=-inf  calFormat='-1'  calUnit=''  calHelp=''  calAccess=1  calFunction=[raptor_xcp_function(gcb) '|' raptor_get_param_eval(gcb, 'paramName') '_Override']
      settings: SourceProductName=Raptor
  wires:
  NOT/1 -> Logical Operator1/2
  raptor_data_read20/1 -> "WH "/2(Voltage input)
  raptor_data_read16/1 -> Compare To Zero/1, Abs/1, Coulomb Counting Algorithm/1(Ampere input)
  raptor_data_read19/1 -> Add3/1
  Gain4/1 -> Switch4/3, Switch1/1
  Divide/1 -> Gain3/1
  raptor_override2/1 -> raptor_data_write8/1
  Add3/1 -> Gain4/1
  "WH "/1(WH Output) -> raptor_override2/1
  raptor_data_read22/1 -> NOT1/1
  raptor_data_read14/1 -> Divide/2
  Gain3/1 -> Switch4/1
  raptor_data_read21/1 -> "WH "/3(WH input)
  Switch4/1 -> raptor_data_write6/1
  Logical Operator1/1 -> NOT2/1, Delay/1(Condition)
  raptor_adjustment2/1 -> Switch4/2
  Constant1/1 -> Delay/2(TimeCount)
  NOT2/1 -> Latch/2(Reset)
  raptor_data_read17/1 -> Divide/1, Switch1/3, Compare To Constant1/1
  Delay/1(Output) -> Latch/1(Latch)
  Latch/1(Output) -> Switch1/2
  raptor_data_read15/1 -> NOT/1
  Compare To Constant1/1 -> Logical Operator1/1
  raptor_data_read18/1 -> Add3/2
  Switch1/1 -> Coulomb Counting Algorithm/2(RC input)
  NOT1/1 -> Logical Operator1/3
  Divide1/1 -> Gain1/1
  raptor_data_read3/1 -> Divide1/1
  raptor_adjustment1/1 -> Divide1/2, raptor_data_write/1
  Gain1/1 -> raptor_data_write7/1
  Abs/1 -> "WH "/1(Ampere input)
  Compare To Zero/1 -> "WH "/Enable

== system EPT/Foreground_TimeBase_5ms/CHG//DCHG_PW_Control/EOC ==
  Delay1 : Subsystem
  EOC_Table : Subsystem
  IsNonNegative : simulink/Logic and Bit Operations/Compare To Zero  relop=>  OutDataTypeStr=boolean
  Latch1 : Subsystem
  Logical Operator : Logic  Inputs=3  AllPortsSameDT=off  OutDataTypeStr=boolean
  Logical Operator1 : Logic  AllPortsSameDT=off  OutDataTypeStr=boolean
  Relational Operator1 : RelationalOperator  OutDataTypeStr=boolean  RndMeth=Simplest
  raptor_adjustment5 : Raptor_lib/Data Storage/raptor_adjustment  paramName='Delay_EOC'  nameSource=Parameter  initValue=300  dataType=double  storage=Calibration  calDispType=Number  calEnum={'False', 'True'}  calGain=1.0  calOffset=0.0  calMax=inf  calMin=-inf  calFormat='-1'  calUnit=''  calHelp=''  calAccess=1  calFunction=raptor_xcp_function(gcb)  calDispHeaders=off  calColHeaders={'Col1' 'Col2' 'Col3'}  calRowHeaders={'Row1' 'Row2' 'Row3'}
      settings: SourceProductName=Raptor
  raptor_data_read1 : Raptor_lib/Data Storage/raptor_data_read  dataName='Flag_HV_Drive_Relay_On'  dataShape=Scalar  idxSource=Input  idxRow=1  idxCol=1
      settings: SourceProductName=Raptor
  raptor_data_read14 : Raptor_lib/Data Storage/raptor_data_read  dataName='Fault_Reset_Trigger'  dataShape=Scalar  idxSource=Input  idxRow=1  idxCol=1
      settings: SourceProductName=Raptor
  raptor_data_read4 : Raptor_lib/Data Storage/raptor_data_read  dataName='Flag_CHG_Mode'  dataShape=Scalar  idxSource=Input  idxRow=1  idxCol=1
      settings: SourceProductName=Raptor
  raptor_data_read6 : Raptor_lib/Data Storage/raptor_data_read  dataName='EPT_BPOBU_CURR'  dataShape=Scalar  idxSource=Input  idxRow=1  idxCol=1
      settings: SourceProductName=Raptor
  raptor_data_read8 : Raptor_lib/Data Storage/raptor_data_read  dataName='Max_CellV'  dataShape=Scalar  idxSource=Input  idxRow=1  idxCol=1
      settings: SourceProductName=Raptor
  raptor_data_write2 : Raptor_lib/Data Storage/raptor_data_write  dataName='Warning_EndOfCharge'  dataShape=Scalar  idxSource=Input Port  idxRow=1  idxCol=1
      settings: SourceProductName=Raptor
  wires:
  EOC_Table/1(CellVoltage) -> Relational Operator1/2
  raptor_data_read8/1 -> Relational Operator1/1
  IsNonNegative/1 -> Logical Operator/2
  raptor_data_read1/1 -> Logical Operator/1
  raptor_data_read6/1 -> IsNonNegative/1
  Relational Operator1/1 -> Logical Operator1/2
  Logical Operator/1 -> Logical Operator1/1
  Logical Operator1/1 -> Delay1/1(Condition)
  Delay1/1(Output) -> Latch1/1(Latch)
  raptor_adjustment5/1 -> Delay1/2(TimeCount)
  raptor_data_read14/1 -> Latch1/2(Reset)
  raptor_data_read4/1 -> Logical Operator/3
  Latch1/1(Output) -> raptor_data_write2/1

== system EPT/Foreground_TimeBase_5ms/CHG//DCHG_PW_Control/EOD ==
  Delay1 : Subsystem
  EOD_Table : Subsystem
  IsNonNegative : simulink/Logic and Bit Operations/Compare To Zero  relop=<  OutDataTypeStr=boolean
  Latch1 : Subsystem
  Logical Operator : Logic  Inputs=3  AllPortsSameDT=off  OutDataTypeStr=boolean
  Logical Operator1 : Logic  AllPortsSameDT=off  OutDataTypeStr=boolean
  Relational Operator : RelationalOperator  Operator=<=  OutDataTypeStr=boolean  RndMeth=Simplest
  raptor_adjustment5 : Raptor_lib/Data Storage/raptor_adjustment  paramName='Delay_EOD'  nameSource=Parameter  initValue=250  dataType=double  storage=Calibration  calDispType=Number  calEnum={'False', 'True'}  calGain=1.0  calOffset=0.0  calMax=inf  calMin=-inf  calFormat='-1'  calUnit=''  calHelp=''  calAccess=1  calFunction=raptor_xcp_function(gcb)  calDispHeaders=off  calColHeaders={'Col1' 'Col2' 'Col3'}  calRowHeaders={'Row1' 'Row2' 'Row3'}
      settings: SourceProductName=Raptor
  raptor_data_read1 : Raptor_lib/Data Storage/raptor_data_read  dataName='Flag_HV_Drive_Relay_On'  dataShape=Scalar  idxSource=Input  idxRow=1  idxCol=1
      settings: SourceProductName=Raptor
  raptor_data_read10 : Raptor_lib/Data Storage/raptor_data_read  dataName='Min_CellV'  dataShape=Scalar  idxSource=Input  idxRow=1  idxCol=1
      settings: SourceProductName=Raptor
  raptor_data_read14 : Raptor_lib/Data Storage/raptor_data_read  dataName='Fault_Reset_Trigger'  dataShape=Scalar  idxSource=Input  idxRow=1  idxCol=1
      settings: SourceProductName=Raptor
  raptor_data_read3 : Raptor_lib/Data Storage/raptor_data_read  dataName='Flag_Drive_Mode'  dataShape=Scalar  idxSource=Input  idxRow=1  idxCol=1
      settings: SourceProductName=Raptor
  raptor_data_read6 : Raptor_lib/Data Storage/raptor_data_read  dataName='EPT_BPOBU_CURR'  dataShape=Scalar  idxSource=Input  idxRow=1  idxCol=1
      settings: SourceProductName=Raptor
  raptor_data_write6 : Raptor_lib/Data Storage/raptor_data_write  dataName='Warning_EndOfDischarge'  dataShape=Scalar  idxSource=Input Port  idxRow=1  idxCol=1
      settings: SourceProductName=Raptor
  wires:
  raptor_data_read10/1 -> Relational Operator/1
  EOD_Table/1(CellVoltage) -> Relational Operator/2
  Logical Operator/1 -> Logical Operator1/1
  raptor_data_read6/1 -> IsNonNegative/1
  raptor_data_read1/1 -> Logical Operator/1
  IsNonNegative/1 -> Logical Operator/2
  Relational Operator/1 -> Logical Operator1/2
  Latch1/1(Output) -> raptor_data_write6/1
  raptor_adjustment5/1 -> Delay1/2(TimeCount)
  Delay1/1(Output) -> Latch1/1(Latch)
  Logical Operator1/1 -> Delay1/1(Condition)
  raptor_data_read14/1 -> Latch1/2(Reset)
  raptor_data_read3/1 -> Logical Operator/3

== system EPT/Foreground_TimeBase_5ms/CHG//DCHG_PW_Control/Enhanced Coulomb Counting Algorithm ==
  Add4 : Sum  Inputs=+-
  Add5 : Sum
  Coulomb Counting : Subsystem
  Delay2 : Delay  DelayLength=1
  Divide1 : Product  Inputs=**
  Divide2 : Product  Inputs=*/
  Divide3 : Product  Inputs=**
  Divide4 : Product  Inputs=**
  Divide8 : Product  Inputs=*/
  Gain : Gain  Gain=100
  Gain1 : Gain  Gain=100
  Init Enhanced Coulomb Counting Algorithm : Subsystem
  Switch5 : Switch  Criteria=u2 > Threshold
  Switch6 : Switch  Criteria=u2 > Threshold
  raptor_adjustment : Raptor_lib/Data Storage/raptor_adjustment  paramName='Cal_Init_Enhance_Coulomb_Counting_Algorithm'  nameSource=Parameter  initValue=0.00  dataType=boolean  storage=Calibration  calDispType=Number  calEnum={'False', 'True'}  calGain=1.0  calOffset=0.0  calMax=inf  calMin=-inf  calFormat='-1'  calUnit=''  calHelp=''  calAccess=1  calFunction=raptor_xcp_function(gcb)  calDispHeaders=off  calColHeaders={'Col1' 'Col2' 'Col3'}  calRowHeaders={'Row1' 'Row2' 'Row3'}
      settings: SourceProductName=Raptor
  raptor_adjustment1 : Raptor_lib/Data Storage/raptor_adjustment  paramName='Cal_BP_OBU_AH_Def'  nameSource=Parameter  initValue=135  dataType=uint8  storage=Calibration  calDispType=Number  calEnum={'False', 'True'}  calGain=1.0  calOffset=0.0  calMax=inf  calMin=-inf  calFormat='-1'  calUnit=''  calHelp=''  calAccess=1  calFunction=raptor_xcp_function(gcb)  calDispHeaders=off  calColHeaders={'Col1' 'Col2' 'Col3'}  calRowHeaders={'Row1' 'Row2' 'Row3'}
      settings: SourceProductName=Raptor
  raptor_data_read1 : Raptor_lib/Data Storage/raptor_data_read  dataName='New_SOH'  dataShape=Scalar  idxSource=Input  idxRow=1  idxCol=1
      settings: SourceProductName=Raptor
  raptor_data_read19 : Raptor_lib/Data Storage/raptor_data_read  dataName='EPT_BPOBU_CURR'  dataShape=Scalar  idxSource=Input  idxRow=1  idxCol=1
      settings: SourceProductName=Raptor
  raptor_data_read2 : Raptor_lib/Data Storage/raptor_data_read  dataName='Warning_EndOfCharge'  dataShape=Scalar  idxSource=Input  idxRow=1  idxCol=1
      settings: SourceProductName=Raptor
  raptor_data_read22 : Raptor_lib/Data Storage/raptor_data_read  dataName='DOD_t0'  dataShape=Scalar  idxSource=Input  idxRow=1  idxCol=1
      settings: SourceProductName=Raptor
  raptor_data_read3 : Raptor_lib/Data Storage/raptor_data_read  dataName='Warning_EndOfDischarge'  dataShape=Scalar  idxSource=Input  idxRow=1  idxCol=1
      settings: SourceProductName=Raptor
  raptor_data_read4 : Raptor_lib/Data Storage/raptor_data_read  dataName='SOH'  dataShape=Scalar  idxSource=Input  idxRow=1  idxCol=1
      settings: SourceProductName=Raptor
  raptor_data_read6 : Raptor_lib/Data Storage/raptor_data_read  dataName='EPT_BPOBU_AH_DEF'  dataShape=Scalar  idxSource=Input  idxRow=1  idxCol=1
      settings: SourceProductName=Raptor
  raptor_data_write : Raptor_lib/Data Storage/raptor_data_write  dataName='EPT_BPOBU_AH_DEF'  dataShape=Scalar  idxSource=Input Port  idxRow=1  idxCol=1
      settings: SourceProductName=Raptor
  raptor_data_write1 : Raptor_lib/Data Storage/raptor_data_write  dataName='EPT_BPOBU_SOC'  dataShape=Scalar  idxSource=Input Port  idxRow=1  idxCol=1
      settings: SourceProductName=Raptor
  raptor_data_write10 : Raptor_lib/Data Storage/raptor_data_write  dataName='DOD_t'  dataShape=Scalar  idxSource=Input Port  idxRow=1  idxCol=1
      settings: SourceProductName=Raptor
  raptor_data_write11 : Raptor_lib/Data Storage/raptor_data_write  dataName='New_SOH'  dataShape=Scalar  idxSource=Input Port  idxRow=1  idxCol=1
      settings: SourceProductName=Raptor
  raptor_data_write2 : Raptor_lib/Data Storage/raptor_data_write  dataName='EPT_BPOBU_FCCAP'  dataShape=Scalar  idxSource=Input Port  idxRow=1  idxCol=1
      settings: SourceProductName=Raptor
  raptor_data_write3 : Raptor_lib/Data Storage/raptor_data_write  dataName='EPT_BPOBU_SOA'  dataShape=Scalar  idxSource=Input Port  idxRow=1  idxCol=1
      settings: SourceProductName=Raptor
  raptor_data_write4 : Raptor_lib/Data Storage/raptor_data_write  dataName='EPT_BPOBU_RCAP'  dataShape=Scalar  idxSource=Input Port  idxRow=1  idxCol=1
      settings: SourceProductName=Raptor
  raptor_data_write5 : Raptor_lib/Data Storage/raptor_data_write  dataName='SOC'  dataShape=Scalar  idxSource=Input Port  idxRow=1  idxCol=1
      settings: SourceProductName=Raptor
  raptor_data_write9 : Raptor_lib/Data Storage/raptor_data_write  dataName='Delta_DOD'  dataShape=Scalar  idxSource=Input Port  idxRow=1  idxCol=1
      settings: SourceProductName=Raptor
  wires:
  raptor_adjustment/1 -> Init Enhanced Coulomb Counting Algorithm/Enable
  raptor_data_read2/1 -> [EOC]
  raptor_data_read3/1 -> [EOD]
  raptor_data_read4/1 -> Add4/1, Switch5/3
  Delay2/1 -> Coulomb Counting/2(Ah Input)
  Divide8/1 -> Gain1/1
  Gain1/1 -> raptor_data_write9/1, Add5/1
  Coulomb Counting/1(Ah Output) -> Divide8/1, Delay2/1
  raptor_data_read19/1 -> Coulomb Counting/1(Ib)
  Add4/1 -> raptor_data_write5/1, [SOC], Switch6/1
  Switch5/1 -> Switch6/3
  Add5/1 -> Switch5/1, raptor_data_write10/1, Add4/2
  Switch6/1 -> raptor_data_write11/1
  raptor_data_read6/1 -> Divide1/1, Divide8/2, Divide4/1
  [EOD] -> Switch5/2
  [EOC] -> Switch6/2
  raptor_data_read22/1 -> Add5/2
  raptor_data_read1/1 -> raptor_data_write3/1, Divide4/2
  [SOC] -> Divide1/2
  Divide1/1 -> Divide2/1
  Divide4/1 -> Divide2/2, Divide3/2, raptor_data_write2/1
  Divide2/1 -> Gain/1
  Gain/1 -> Divide3/1, raptor_data_write1/1
  Divide3/1 -> raptor_data_write4/1
  raptor_adjustment1/1 -> raptor_data_write/1

== system EPT/Foreground_TimeBase_5ms/CHG//DCHG_PW_Control/Enhanced Coulomb Counting Algorithm Backup ==
  Add1 : Sum  Inputs=+-
  Add2 : Sum
  Coulomb Counting1 : Subsystem
  Delay1 : Delay  DelayLength=1
  Divide6 : Product  Inputs=*/
  Divide8 : Product  Inputs=**
  Gain1 : Gain  Gain=0.01
  Gain3 : Gain  Gain=100
  Switch3 : Switch  Criteria=u2 > Threshold
  Switch4 : Switch  Criteria=u2 > Threshold
  raptor_data_read1 : Raptor_lib/Data Storage/raptor_data_read  dataName='Crated'  dataShape=Scalar  idxSource=Input  idxRow=1  idxCol=1
      settings: SourceProductName=Raptor
  raptor_data_read15 : Raptor_lib/Data Storage/raptor_data_read  dataName='SOH'  dataShape=Scalar  idxSource=Input  idxRow=1  idxCol=1
      settings: SourceProductName=Raptor
  raptor_data_read19 : Raptor_lib/Data Storage/raptor_data_read  dataName='EPT_BPOBU_CURR'  dataShape=Scalar  idxSource=Input  idxRow=1  idxCol=1
      settings: SourceProductName=Raptor
  raptor_data_read2 : Raptor_lib/Data Storage/raptor_data_read  dataName='Warning_EndOfCharge'  dataShape=Scalar  idxSource=Input  idxRow=1  idxCol=1
      settings: SourceProductName=Raptor
  raptor_data_read22 : Raptor_lib/Data Storage/raptor_data_read  dataName='DOD_t0'  dataShape=Scalar  idxSource=Input  idxRow=1  idxCol=1
      settings: SourceProductName=Raptor
  raptor_data_read3 : Raptor_lib/Data Storage/raptor_data_read  dataName='Warning_EndOfDischarge'  dataShape=Scalar  idxSource=Input  idxRow=1  idxCol=1
      settings: SourceProductName=Raptor
  raptor_data_write10 : Raptor_lib/Data Storage/raptor_data_write  dataName='DOD_t'  dataShape=Scalar  idxSource=Input Port  idxRow=1  idxCol=1
      settings: SourceProductName=Raptor
  raptor_data_write11 : Raptor_lib/Data Storage/raptor_data_write  dataName='New_SOH'  dataShape=Scalar  idxSource=Input Port  idxRow=1  idxCol=1
      settings: SourceProductName=Raptor
  raptor_data_write12 : Raptor_lib/Data Storage/raptor_data_write  dataName='Cmax'  dataShape=Scalar  idxSource=Input Port  idxRow=1  idxCol=1
      settings: SourceProductName=Raptor
  raptor_data_write7 : Raptor_lib/Data Storage/raptor_data_write  dataName='SOC'  dataShape=Scalar  idxSource=Input Port  idxRow=1  idxCol=1
      settings: SourceProductName=Raptor
  raptor_data_write9 : Raptor_lib/Data Storage/raptor_data_write  dataName='Delta_DOD'  dataShape=Scalar  idxSource=Input Port  idxRow=1  idxCol=1
      settings: SourceProductName=Raptor
  wires:
  [EOD] -> Switch3/2
  [EOC] -> Switch4/2
  raptor_data_read3/1 -> [EOD]
  raptor_data_read2/1 -> [EOC]
  Add1/1 -> raptor_data_write7/1, Switch4/1
  Gain1/1 -> raptor_data_write12/1
  raptor_data_read15/1 -> Add1/1, Switch3/3, Divide8/1
  raptor_data_read19/1 -> Coulomb Counting1/1(Ib)
  raptor_data_read1/1 -> Divide8/2, Divide6/2
  Divide8/1 -> Gain1/1
  Divide6/1 -> Gain3/1
  Add2/1 -> raptor_data_write10/1, Switch3/1, Add1/2
  Gain3/1 -> raptor_data_write9/1, Add2/1
  Coulomb Counting1/1(Ah Output) -> Divide6/1, Delay1/1
  Delay1/1 -> Coulomb Counting1/2(Ah Input)
  Switch4/1 -> raptor_data_write11/1
  raptor_data_read22/1 -> Add2/2
  Switch3/1 -> Switch4/3

== system EPT/Foreground_TimeBase_5ms/CHG//DCHG_PW_Control/Maximum allowable Regen torque ==
  Iregen_con : Inport
  Abs : Abs
  Abs1 : Abs
  Compare To Constant : simulink/Logic and Bit Operations/Compare To Constant  relop=<=  const=5  OutDataTypeStr=boolean
  Constant : Constant
  Data Type Conversion : DataTypeConversion
  Data Type Conversion1 : DataTypeConversion
  Delay : Delay  DelayLength=1  InitialCondition=0
  Divide : Product  Inputs=*/
  Gain1 : Gain  Gain=0.01
  Gain2 : Gain  Gain=9.54805
  Product : Product  Inputs=3
  Saturation : Saturate  UpperLimit=150  LowerLimit=0
  Switch : Switch  Criteria=u2 > Threshold
  raptor_data_read1 : Raptor_lib/Data Storage/raptor_data_read  dataName='EPT_BPOBU_VOLT'  dataShape=Scalar  idxSource=Input  idxRow=1  idxCol=1
      settings: SourceProductName=Raptor
  raptor_data_read2 : Raptor_lib/Data Storage/raptor_data_read  dataName='Read_Motor_Speed'  dataShape=Scalar  idxSource=Input  idxRow=1  idxCol=1
      settings: SourceProductName=Raptor
  raptor_data_write : Raptor_lib/Data Storage/raptor_data_write  dataName='EPT_MAX_REG_TRQ'  dataShape=Scalar  idxSource=Input Port  idxRow=1  idxCol=1
      settings: SourceProductName=Raptor
  raptor_measurement1 : Raptor_lib/Data Storage/raptor_measurement  paramName='Regen_efficiency'  nameSource=Parameter  calDispType=Number  calEnum={'False', 'True'}  calGain=1.0  calOffset=0.0  calMax=inf  calMin=-inf  calFormat='-1'  calUnit=''  calHelp=''  calAccess=1  calFunction=raptor_xcp_function(gcb)  calVisible=on
      settings: SourceProductName=Raptor
  raptor_table_2d : Raptor_lib/Table Lookup/raptor_table_2d  dataName='Regen_Efficiency'  initValue=|  dataType=double  storage=Calibration  initValueX="[0\t300\t600\t1200\t1800\t2400\t3000\t3600\t4200\t4800\t5400\t6000]"  initValueY="[0\t7.5\t15\t30\t45\t60\t75\t90\t105\t120\t135\t150]"  dataTypeXY=double  storageXY=Calibration  calVisible=on  showTable=off  calGain=1.0  calOffset=0.0  calMax=Inf  calMin=-Inf  calFormat='-1'  calUnit=''  calHelp=''  showBreakpointX=off  dataNameX=[]  calGainX=1.0  calOffsetX=0.0  calMaxX=Inf  calMinX=-Inf  calFormatX='-1'  calUnitX=''  calHelpX=''  showBreakpointY=off  dataNameY=[]  calGainY=1.0  calOffsetY=0.0  calMaxY=Inf  calMinY=-Inf  calFormatY='-1'  calUnitY=''  calHelpY=''  calAccess=1  calFunction=raptor_xcp_function(gcb)  measureEnable=off  mName=[raptor_get_param_eval(gcb,'dataName'), '_Output']
      | [50	50	50	50	50	50	50	50	50	50	50	50;
      | 55	60	62.5	65	70	72.5	75	77.5	77.5	75	72.5	70;
      | 57.5	62.5	65	70	77.5	80	80	82.5	82.5	80	77.5	75;
      | 57.5	65	67.5	72.5	80	82.5	85	85	85	85	85	82.5;
      | 60	67.5	70	80	85	85	87.5	87.5	87.5	87.5	87.5	85;
      | 60	67.5	72.5	82.5	87.5	87.5	90	90	90	87.5	85	82.5;
      | 62.5	70	75	82.5	87.5	90	90	87.5	85	82.5	82.5	80;
      | 62.5	72.5	77.5	85	90	90	87.5	85	82.5	80	80	77.5;
      | 65	72.5	77.5	85	90	90	85	82.5	80	77.5	80	75;
      | 65	72.5	75	82.5	90	87.5	82.5	80	80	75	77.5	72.5;
      | 67.5	70	75	82.5	87.5	85	82.5	80	77.5	75	75	70;
      | 67.5	70	72.5	80	85	82.5	77.5	75	77.5	72.5	75	70;]
      settings: SourceProductName=Raptor
  wires:
  Data Type Conversion1/1 -> raptor_data_write/1
  Delay/1 -> raptor_table_2d/1
  Divide/1 -> Saturation/1
  Data Type Conversion/1 -> raptor_table_2d/2, Compare To Constant/1, Switch/3
  Abs1/1 -> Data Type Conversion/1
  Gain1/1 -> Product/1
  raptor_table_2d/1 -> Gain1/1, raptor_measurement1/1
  Saturation/1 -> Data Type Conversion1/1, Delay/1
  Constant/1 -> Switch/1
  Compare To Constant/1 -> Switch/2
  raptor_data_read2/1 -> Abs1/1
  raptor_data_read1/1 -> Product/2
  Abs/1 -> Product/3
  Switch/1 -> Divide/2
  Product/1 -> Gain2/1
  Iregen_con/1 -> Abs/1
  Gain2/1 -> Divide/1
